simulink model "verify"  (R2018a)
settings: Solver=ode4  StartTime=0.0  StopTime=10.0  FixedStep=0.01  RelTol=1e-3
settings Model: Creator=lenovo  LastModifiedBy=lenovo

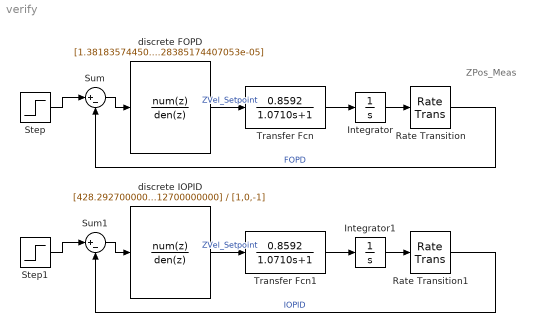
== system verify ==
  note: ZPos_Meas
  Integrator : Integrator
  Integrator1 : Integrator
  Rate Transition : RateTransition  OutPortSampleTime=0.01
  Rate Transition1 : RateTransition  OutPortSampleTime=0.01
  Step : Step  SampleTime=0.01
  Step1 : Step  SampleTime=0.01
  Sum : Sum  Inputs=|+-
  Sum1 : Sum  Inputs=|+-
  Transfer Fcn : TransferFcn  Numerator=[0.8592]  Denominator=[1.0710 1]
  Transfer Fcn1 : TransferFcn  Numerator=[0.8592]  Denominator=[1.0710 1]
  discrete FOPD : DiscreteTransferFcn  Numerator=[1.38183574450685,-4.65873433127261,5.91849466326920,-3.45032645121382,0.877255899520245,-0.0684747220777590]  Denominator=[0.00924006359793744,-0.0207875447450158,0.0147933870749008,-0.00294076599412286,-0.000345393194545685,7.28385174407053e-05]  SampleTime=0.01
  discrete IOPID : DiscreteTransferFcn  Numerator=[428.292700000000,-851.994600000000,423.712700000000]  Denominator=[1,0,-1]  SampleTime=0.01
  wires:
  Step/1 -> Sum/1
  Sum/1 -> discrete FOPD/1
  discrete FOPD/1 -> Transfer Fcn/1  "ZVel_Setpoint"
  Transfer Fcn/1 -> Integrator/1
  Integrator/1 -> Rate Transition/1
  Rate Transition/1 -> Sum/2  "FOPD"
  Step1/1 -> Sum1/1
  discrete IOPID/1 -> Transfer Fcn1/1  "ZVel_Setpoint"
  Sum1/1 -> discrete IOPID/1
  Transfer Fcn1/1 -> Integrator1/1
  Rate Transition1/1 -> Sum1/2  "IOPID"
  Integrator1/1 -> Rate Transition1/1
